simulink library "quat_kinematics_lib"  (R2018b)
settings: Solver=VariableStepAuto  StartTime=0.0  StopTime=10.0  RelTol=1e-3
undefined symbols (not defined in the file or in its folder): simParams
libraries: sharedutil x1
settings Model: Creator=taylorreynolds  LastModifiedBy=Taylor

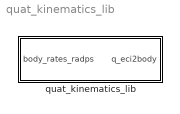
== system quat_kinematics_lib ==
  quat_kinematics_lib : Subsystem

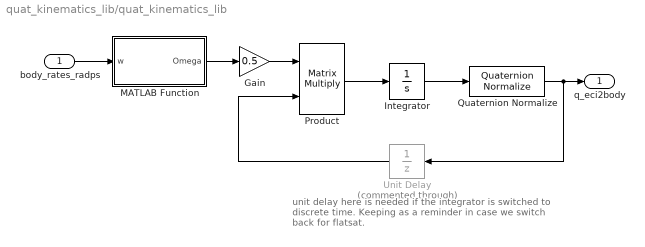
== system quat_kinematics_lib/quat_kinematics_lib ==
  note: unit delay here is needed if the integrator is
      | switched to discrete time. Keeping as a reminder
      | in case we switch back for flatsat.
  body_rates_radps : Inport
  Gain : Gain  Gain=0.5
  Integrator : Integrator  InitialCondition=simParams.initialConditions.q_eci2body
  MATLAB Function : MATLAB Function  TreatAsAtomicUnit=on
  Product : Product  Multiplication=Matrix(*)
  Quaternion Normalize : sharedutil/Quaternion Normalize  aMode=aMode
      settings: SourceProductName=Aerospace Blockset  SourceProductBaseCode=AE
  Unit Delay : UnitDelay  Commented=through  InitialCondition=simParams.initialConditions.q_eci2body  SampleTime=-1
  q_eci2body : Outport
  wires:
  Quaternion Normalize/1 -> q_eci2body/1, Unit Delay/1
  Integrator/1 -> Quaternion Normalize/1
  body_rates_radps/1 -> MATLAB Function/1(w)
  MATLAB Function/1(Omega) -> Gain/1
  Product/1 -> Integrator/1
  Gain/1 -> Product/1
  Unit Delay/1 -> Product/2

== matlab function quat_kinematics_lib/MATLAB Function ==
  data: w input; Omega output
function Omega = q_skew_star(w)
%#codegen
Omega = [ 0.0,  -w(1), -w(2), -w(3);
          w(1),  0.0,   w(3), -w(2);
          w(2), -w(3),  0.0,   w(1);
          w(3),  w(2), -w(1),  0.0 ];
end
